simulink model "TST_RngMod_TrqFrcCalc"  (R2016b)
settings: Solver=FixedStepDiscrete  StartTime=0.0  StopTime=simTime  FixedStep=sampleTime  RelTol=1e-3
values from neighbouring files (symbols this model uses):
  testCase = 1    [initTST_RngMod_TrqFrcCalc_001.m]    (also in initTST_RngMod_TrqFrcCalc_002.m = 2; initTST_RngMod_TrqFrcCalc_003.m = 3)
libraries: simulink x4
settings Model: Creator=guofang02  LastModifiedBy=guofang02
settings ConfigComp: CovHTMLOptions=-sRT=0  CovHtmlReporting=on  CovSaveCumulativeToWorkspaceVar=on  CovCumulativeVarName=RngMod_TrqFrcCalc_covCumulativeData  CovCumulativeReport=on  CovShowResultsExplorer=off

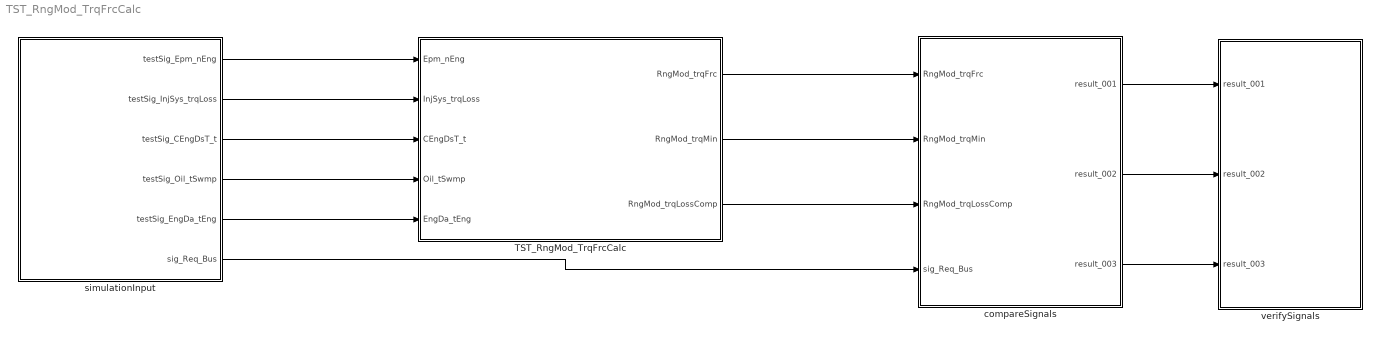
== system TST_RngMod_TrqFrcCalc ==
  TST_RngMod_TrqFrcCalc : Subsystem
  compareSignals : Subsystem
  simulationInput : Subsystem
  verifySignals : Subsystem
  wires:
  simulationInput/1(testSig_Epm_nEng) -> TST_RngMod_TrqFrcCalc/1(Epm_nEng)
  simulationInput/2(testSig_InjSys_trqLoss) -> TST_RngMod_TrqFrcCalc/2(InjSys_trqLoss)
  simulationInput/3(testSig_CEngDsT_t) -> TST_RngMod_TrqFrcCalc/3(CEngDsT_t)
  simulationInput/4(testSig_Oil_tSwmp) -> TST_RngMod_TrqFrcCalc/4(Oil_tSwmp)
  simulationInput/5(testSig_EngDa_tEng) -> TST_RngMod_TrqFrcCalc/5(EngDa_tEng)
  TST_RngMod_TrqFrcCalc/1(RngMod_trqFrc) -> compareSignals/1(RngMod_trqFrc)
  TST_RngMod_TrqFrcCalc/2(RngMod_trqMin) -> compareSignals/2(RngMod_trqMin)
  TST_RngMod_TrqFrcCalc/3(RngMod_trqLossComp) -> compareSignals/3(RngMod_trqLossComp)
  simulationInput/6(sig_Req_Bus) -> compareSignals/4(sig_Req_Bus)
  compareSignals/1(result_001) -> verifySignals/1(result_001)
  compareSignals/2(result_002) -> verifySignals/2(result_002)
  compareSignals/3(result_003) -> verifySignals/3(result_003)

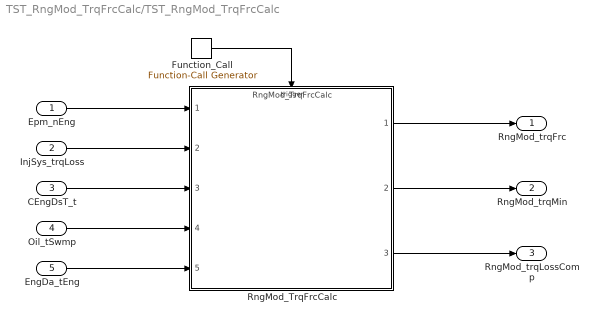
== system TST_RngMod_TrqFrcCalc/TST_RngMod_TrqFrcCalc ==
  Epm_nEng : Inport
  InjSys_trqLoss : Inport  Port=2
  CEngDsT_t : Inport  Port=3
  Oil_tSwmp : Inport  Port=4
  EngDa_tEng : Inport  Port=5
  Function_Call : simulink/Ports & Subsystems/Function-Call Generator  sample_time=sampleTime  numberOfIterations=1
  RngMod_TrqFrcCalc : ModelReference  ModelNameDialog=RngMod_TrqFrcCalc  SimulationMode=Normal  ModelReferenceVersion=1.4  TriggerPortName=function  TriggerPortTriggerType=function-call  TriggerPortStatesWhenEnabling=held
  RngMod_trqFrc : Outport
  RngMod_trqMin : Outport  Port=2
  RngMod_trqLossComp : Outport  Port=3
  wires:
  Function_Call/1 -> RngMod_TrqFrcCalc/Trigger
  Epm_nEng/1 -> RngMod_TrqFrcCalc/1
  InjSys_trqLoss/1 -> RngMod_TrqFrcCalc/2
  CEngDsT_t/1 -> RngMod_TrqFrcCalc/3
  Oil_tSwmp/1 -> RngMod_TrqFrcCalc/4
  EngDa_tEng/1 -> RngMod_TrqFrcCalc/5
  RngMod_TrqFrcCalc/1 -> RngMod_trqFrc/1
  RngMod_TrqFrcCalc/2 -> RngMod_trqMin/1
  RngMod_TrqFrcCalc/3 -> RngMod_trqLossComp/1

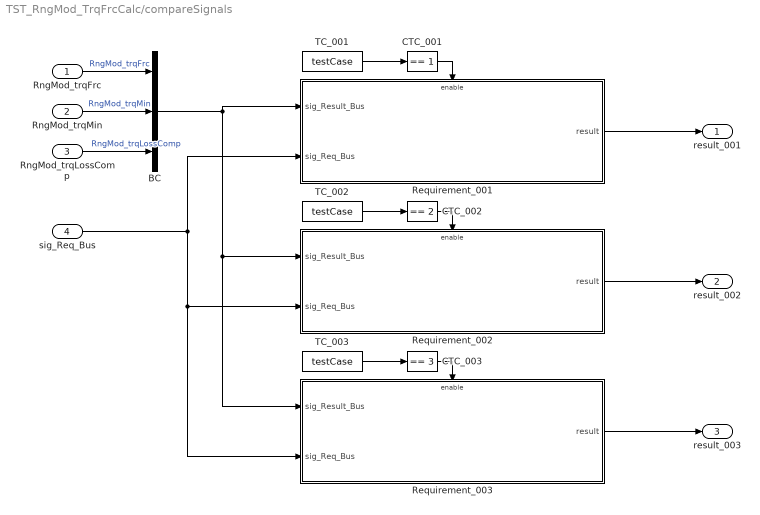
== system TST_RngMod_TrqFrcCalc/compareSignals ==
  RngMod_trqFrc : Inport
  RngMod_trqMin : Inport  Port=2
  RngMod_trqLossComp : Inport  Port=3
  sig_Req_Bus : Inport  Port=4
  BC : BusCreator  Inputs=3
  CTC_001 : simulink/Logic and Bit Operations/Compare To Constant  relop===  const=1  OutDataTypeStr=boolean
  CTC_002 : simulink/Logic and Bit Operations/Compare To Constant  relop===  const=2  OutDataTypeStr=boolean
  CTC_003 : simulink/Logic and Bit Operations/Compare To Constant  relop===  const=3  OutDataTypeStr=boolean
  Requirement_001 : Subsystem
  Requirement_002 : Subsystem
  Requirement_003 : Subsystem
  TC_001 : Constant  Value=testCase
  TC_002 : Constant  Value=testCase
  TC_003 : Constant  Value=testCase
  result_001 : Outport
  result_002 : Outport  Port=2
  result_003 : Outport  Port=3
  wires:
  RngMod_trqFrc/1 -> BC/1  "RngMod_trqFrc"
  RngMod_trqMin/1 -> BC/2  "RngMod_trqMin"
  RngMod_trqLossComp/1 -> BC/3  "RngMod_trqLossComp"
  TC_001/1 -> CTC_001/1
  CTC_001/1 -> Requirement_001/Enable
  sig_Req_Bus/1 -> Requirement_002/2(sig_Req_Bus), Requirement_003/2(sig_Req_Bus), Requirement_001/2(sig_Req_Bus)
  BC/1 -> Requirement_002/1(sig_Result_Bus), Requirement_003/1(sig_Result_Bus), Requirement_001/1(sig_Result_Bus)
  Requirement_001/1(result) -> result_001/1
  TC_002/1 -> CTC_002/1
  CTC_002/1 -> Requirement_002/Enable
  Requirement_002/1(result) -> result_002/1
  TC_003/1 -> CTC_003/1
  CTC_003/1 -> Requirement_003/Enable
  Requirement_003/1(result) -> result_003/1

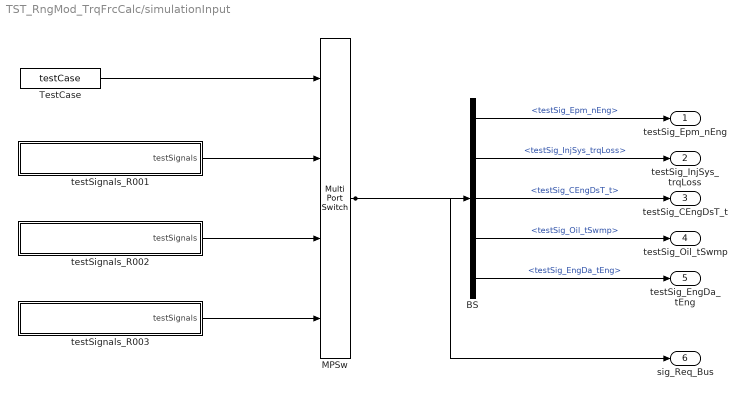
== system TST_RngMod_TrqFrcCalc/simulationInput ==
  BS : BusSelector  OutputSignals=testSig_Epm_nEng,testSig_InjSys_trqLoss,testSig_CEngDsT_t,testSig_Oil_tSwmp,testSig_EngDa_tEng
  MPSw : MultiPortSwitch  SaturateOnIntegerOverflow=on  InputSameDT=on
  TestCase : Constant  Value=testCase
  testSignals_R001 : Subsystem
  testSignals_R002 : Subsystem
  testSignals_R003 : Subsystem
  testSig_Epm_nEng : Outport
  testSig_InjSys_trqLoss : Outport  Port=2
  testSig_CEngDsT_t : Outport  Port=3
  testSig_Oil_tSwmp : Outport  Port=4
  testSig_EngDa_tEng : Outport  Port=5
  sig_Req_Bus : Outport  Port=6
  wires:
  BS/1 -> testSig_Epm_nEng/1  "<testSig_Epm_nEng>"
  BS/2 -> testSig_InjSys_trqLoss/1  "<testSig_InjSys_trqLoss>"
  BS/3 -> testSig_CEngDsT_t/1  "<testSig_CEngDsT_t>"
  BS/4 -> testSig_Oil_tSwmp/1  "<testSig_Oil_tSwmp>"
  BS/5 -> testSig_EngDa_tEng/1  "<testSig_EngDa_tEng>"
  MPSw/1 -> BS/1, sig_Req_Bus/1
  TestCase/1 -> MPSw/1
  testSignals_R001/1(testSignals) -> MPSw/2
  testSignals_R002/1(testSignals) -> MPSw/3
  testSignals_R003/1(testSignals) -> MPSw/4

== system TST_RngMod_TrqFrcCalc/verifySignals ==
  result_001 : Inport
  result_002 : Inport  Port=2
  result_003 : Inport  Port=3
  Assertion_001 : Assertion  Enabled=off
  Assertion_002 : Assertion  Enabled=off
  Assertion_003 : Assertion
  wires:
  result_001/1 -> Assertion_001/1
  result_002/1 -> Assertion_002/1
  result_003/1 -> Assertion_003/1

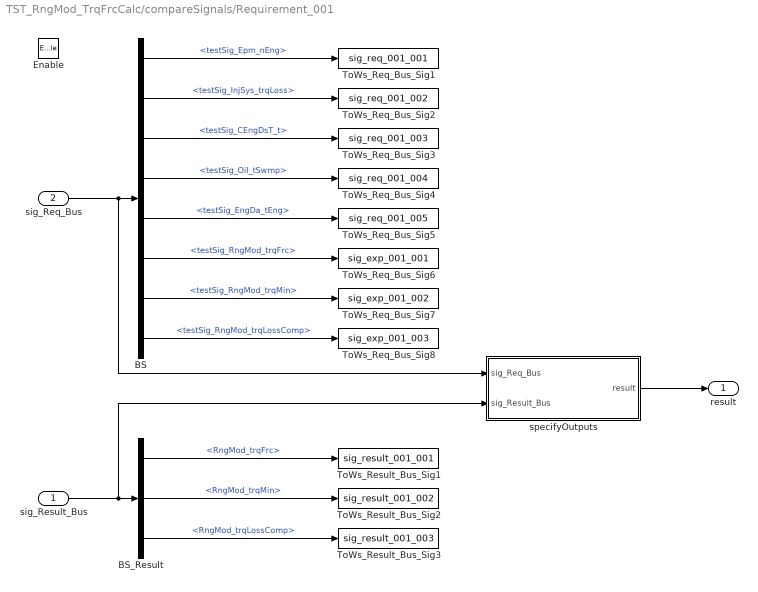
== system TST_RngMod_TrqFrcCalc/compareSignals/Requirement_001 ==
  sig_Result_Bus : Inport
  sig_Req_Bus : Inport  Port=2
  Enable : EnablePort
  BS : BusSelector  OutputSignals=testSig_Epm_nEng,testSig_InjSys_trqLoss,testSig_CEngDsT_t,testSig_Oil_tSwmp,testSig_EngDa_tEng,testSig_RngMod_trqFrc,testSig_RngMod_trqMin,testSig_RngMod_trqLossComp
  BS_Result : BusSelector  OutputSignals=RngMod_trqFrc,RngMod_trqMin,RngMod_trqLossComp
  ToWs_Req_Bus_Sig1 : ToWorkspace  VariableName=sig_req_001_001  SaveFormat=Structure With Time
  ToWs_Req_Bus_Sig2 : ToWorkspace  VariableName=sig_req_001_002  SaveFormat=Structure With Time
  ToWs_Req_Bus_Sig3 : ToWorkspace  VariableName=sig_req_001_003  SaveFormat=Structure With Time
  ToWs_Req_Bus_Sig4 : ToWorkspace  VariableName=sig_req_001_004  SaveFormat=Structure With Time
  ToWs_Req_Bus_Sig5 : ToWorkspace  VariableName=sig_req_001_005  SaveFormat=Structure With Time
  ToWs_Req_Bus_Sig6 : ToWorkspace  VariableName=sig_exp_001_001  SaveFormat=Structure With Time
  ToWs_Req_Bus_Sig7 : ToWorkspace  VariableName=sig_exp_001_002  SaveFormat=Structure With Time
  ToWs_Req_Bus_Sig8 : ToWorkspace  VariableName=sig_exp_001_003  SaveFormat=Structure With Time
  ToWs_Result_Bus_Sig1 : ToWorkspace  VariableName=sig_result_001_001  SaveFormat=Structure With Time
  ToWs_Result_Bus_Sig2 : ToWorkspace  VariableName=sig_result_001_002  SaveFormat=Structure With Time
  ToWs_Result_Bus_Sig3 : ToWorkspace  VariableName=sig_result_001_003  SaveFormat=Structure With Time
  specifyOutputs : Subsystem
  result : Outport
  wires:
  sig_Req_Bus/1 -> BS/1, specifyOutputs/1(sig_Req_Bus)
  BS/1 -> ToWs_Req_Bus_Sig1/1  "<testSig_Epm_nEng>"
  BS/2 -> ToWs_Req_Bus_Sig2/1  "<testSig_InjSys_trqLoss>"
  BS/3 -> ToWs_Req_Bus_Sig3/1  "<testSig_CEngDsT_t>"
  BS/4 -> ToWs_Req_Bus_Sig4/1  "<testSig_Oil_tSwmp>"
  BS/5 -> ToWs_Req_Bus_Sig5/1  "<testSig_EngDa_tEng>"
  BS/6 -> ToWs_Req_Bus_Sig6/1  "<testSig_RngMod_trqFrc>"
  BS/7 -> ToWs_Req_Bus_Sig7/1  "<testSig_RngMod_trqMin>"
  BS/8 -> ToWs_Req_Bus_Sig8/1  "<testSig_RngMod_trqLossComp>"
  sig_Result_Bus/1 -> BS_Result/1, specifyOutputs/2(sig_Result_Bus)
  BS_Result/1 -> ToWs_Result_Bus_Sig1/1  "<RngMod_trqFrc>"
  BS_Result/2 -> ToWs_Result_Bus_Sig2/1  "<RngMod_trqMin>"
  BS_Result/3 -> ToWs_Result_Bus_Sig3/1  "<RngMod_trqLossComp>"
  specifyOutputs/1(result) -> result/1

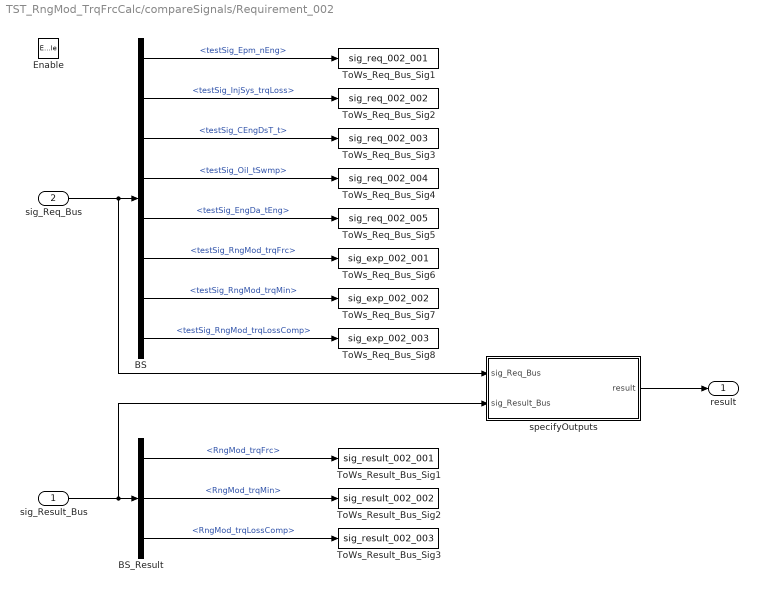
== system TST_RngMod_TrqFrcCalc/compareSignals/Requirement_002 ==
  sig_Result_Bus : Inport
  sig_Req_Bus : Inport  Port=2
  Enable : EnablePort
  BS : BusSelector  OutputSignals=testSig_Epm_nEng,testSig_InjSys_trqLoss,testSig_CEngDsT_t,testSig_Oil_tSwmp,testSig_EngDa_tEng,testSig_RngMod_trqFrc,testSig_RngMod_trqMin,testSig_RngMod_trqLossComp
  BS_Result : BusSelector  OutputSignals=RngMod_trqFrc,RngMod_trqMin,RngMod_trqLossComp
  ToWs_Req_Bus_Sig1 : ToWorkspace  VariableName=sig_req_002_001  SaveFormat=Structure With Time
  ToWs_Req_Bus_Sig2 : ToWorkspace  VariableName=sig_req_002_002  SaveFormat=Structure With Time
  ToWs_Req_Bus_Sig3 : ToWorkspace  VariableName=sig_req_002_003  SaveFormat=Structure With Time
  ToWs_Req_Bus_Sig4 : ToWorkspace  VariableName=sig_req_002_004  SaveFormat=Structure With Time
  ToWs_Req_Bus_Sig5 : ToWorkspace  VariableName=sig_req_002_005  SaveFormat=Structure With Time
  ToWs_Req_Bus_Sig6 : ToWorkspace  VariableName=sig_exp_002_001  SaveFormat=Structure With Time
  ToWs_Req_Bus_Sig7 : ToWorkspace  VariableName=sig_exp_002_002  SaveFormat=Structure With Time
  ToWs_Req_Bus_Sig8 : ToWorkspace  VariableName=sig_exp_002_003  SaveFormat=Structure With Time
  ToWs_Result_Bus_Sig1 : ToWorkspace  VariableName=sig_result_002_001  SaveFormat=Structure With Time
  ToWs_Result_Bus_Sig2 : ToWorkspace  VariableName=sig_result_002_002  SaveFormat=Structure With Time
  ToWs_Result_Bus_Sig3 : ToWorkspace  VariableName=sig_result_002_003  SaveFormat=Structure With Time
  specifyOutputs : Subsystem
  result : Outport
  wires:
  sig_Req_Bus/1 -> BS/1, specifyOutputs/1(sig_Req_Bus)
  BS/1 -> ToWs_Req_Bus_Sig1/1  "<testSig_Epm_nEng>"
  BS/2 -> ToWs_Req_Bus_Sig2/1  "<testSig_InjSys_trqLoss>"
  BS/3 -> ToWs_Req_Bus_Sig3/1  "<testSig_CEngDsT_t>"
  BS/4 -> ToWs_Req_Bus_Sig4/1  "<testSig_Oil_tSwmp>"
  BS/5 -> ToWs_Req_Bus_Sig5/1  "<testSig_EngDa_tEng>"
  BS/6 -> ToWs_Req_Bus_Sig6/1  "<testSig_RngMod_trqFrc>"
  BS/7 -> ToWs_Req_Bus_Sig7/1  "<testSig_RngMod_trqMin>"
  BS/8 -> ToWs_Req_Bus_Sig8/1  "<testSig_RngMod_trqLossComp>"
  sig_Result_Bus/1 -> BS_Result/1, specifyOutputs/2(sig_Result_Bus)
  BS_Result/1 -> ToWs_Result_Bus_Sig1/1  "<RngMod_trqFrc>"
  BS_Result/2 -> ToWs_Result_Bus_Sig2/1  "<RngMod_trqMin>"
  BS_Result/3 -> ToWs_Result_Bus_Sig3/1  "<RngMod_trqLossComp>"
  specifyOutputs/1(result) -> result/1

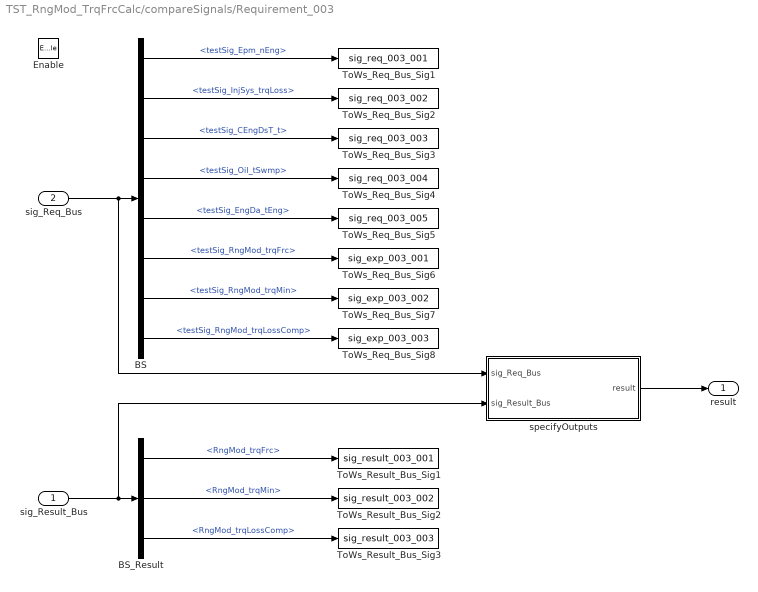
== system TST_RngMod_TrqFrcCalc/compareSignals/Requirement_003 ==
  sig_Result_Bus : Inport
  sig_Req_Bus : Inport  Port=2
  Enable : EnablePort
  BS : BusSelector  OutputSignals=testSig_Epm_nEng,testSig_InjSys_trqLoss,testSig_CEngDsT_t,testSig_Oil_tSwmp,testSig_EngDa_tEng,testSig_RngMod_trqFrc,testSig_RngMod_trqMin,testSig_RngMod_trqLossComp
  BS_Result : BusSelector  OutputSignals=RngMod_trqFrc,RngMod_trqMin,RngMod_trqLossComp
  ToWs_Req_Bus_Sig1 : ToWorkspace  VariableName=sig_req_003_001  SaveFormat=Structure With Time
  ToWs_Req_Bus_Sig2 : ToWorkspace  VariableName=sig_req_003_002  SaveFormat=Structure With Time
  ToWs_Req_Bus_Sig3 : ToWorkspace  VariableName=sig_req_003_003  SaveFormat=Structure With Time
  ToWs_Req_Bus_Sig4 : ToWorkspace  VariableName=sig_req_003_004  SaveFormat=Structure With Time
  ToWs_Req_Bus_Sig5 : ToWorkspace  VariableName=sig_req_003_005  SaveFormat=Structure With Time
  ToWs_Req_Bus_Sig6 : ToWorkspace  VariableName=sig_exp_003_001  SaveFormat=Structure With Time
  ToWs_Req_Bus_Sig7 : ToWorkspace  VariableName=sig_exp_003_002  SaveFormat=Structure With Time
  ToWs_Req_Bus_Sig8 : ToWorkspace  VariableName=sig_exp_003_003  SaveFormat=Structure With Time
  ToWs_Result_Bus_Sig1 : ToWorkspace  VariableName=sig_result_003_001  SaveFormat=Structure With Time
  ToWs_Result_Bus_Sig2 : ToWorkspace  VariableName=sig_result_003_002  SaveFormat=Structure With Time
  ToWs_Result_Bus_Sig3 : ToWorkspace  VariableName=sig_result_003_003  SaveFormat=Structure With Time
  specifyOutputs : Subsystem
  result : Outport
  wires:
  sig_Req_Bus/1 -> BS/1, specifyOutputs/1(sig_Req_Bus)
  BS/1 -> ToWs_Req_Bus_Sig1/1  "<testSig_Epm_nEng>"
  BS/2 -> ToWs_Req_Bus_Sig2/1  "<testSig_InjSys_trqLoss>"
  BS/3 -> ToWs_Req_Bus_Sig3/1  "<testSig_CEngDsT_t>"
  BS/4 -> ToWs_Req_Bus_Sig4/1  "<testSig_Oil_tSwmp>"
  BS/5 -> ToWs_Req_Bus_Sig5/1  "<testSig_EngDa_tEng>"
  BS/6 -> ToWs_Req_Bus_Sig6/1  "<testSig_RngMod_trqFrc>"
  BS/7 -> ToWs_Req_Bus_Sig7/1  "<testSig_RngMod_trqMin>"
  BS/8 -> ToWs_Req_Bus_Sig8/1  "<testSig_RngMod_trqLossComp>"
  sig_Result_Bus/1 -> BS_Result/1, specifyOutputs/2(sig_Result_Bus)
  BS_Result/1 -> ToWs_Result_Bus_Sig1/1  "<RngMod_trqFrc>"
  BS_Result/2 -> ToWs_Result_Bus_Sig2/1  "<RngMod_trqMin>"
  BS_Result/3 -> ToWs_Result_Bus_Sig3/1  "<RngMod_trqLossComp>"
  specifyOutputs/1(result) -> result/1

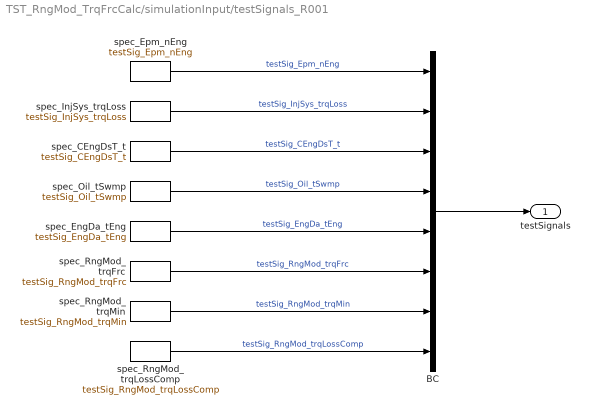
== system TST_RngMod_TrqFrcCalc/simulationInput/testSignals_R001 ==
  BC : BusCreator  Inputs=8
  spec_CEngDsT_t : FromWorkspace  VariableName=testSig_CEngDsT_t  Interpolate=off  OutputAfterFinalValue=Holding final value
  spec_EngDa_tEng : FromWorkspace  VariableName=testSig_EngDa_tEng  Interpolate=off  OutputAfterFinalValue=Holding final value
  spec_Epm_nEng : FromWorkspace  VariableName=testSig_Epm_nEng  Interpolate=off  OutputAfterFinalValue=Holding final value
  spec_InjSys_trqLoss : FromWorkspace  VariableName=testSig_InjSys_trqLoss  Interpolate=off  OutputAfterFinalValue=Holding final value
  spec_Oil_tSwmp : FromWorkspace  VariableName=testSig_Oil_tSwmp  Interpolate=off  OutputAfterFinalValue=Holding final value
  spec_RngMod_trqFrc : FromWorkspace  VariableName=testSig_RngMod_trqFrc  Interpolate=off  OutputAfterFinalValue=Holding final value
  spec_RngMod_trqLossComp : FromWorkspace  VariableName=testSig_RngMod_trqLossComp  Interpolate=off  OutputAfterFinalValue=Holding final value
  spec_RngMod_trqMin : FromWorkspace  VariableName=testSig_RngMod_trqMin  Interpolate=off  OutputAfterFinalValue=Holding final value
  testSignals : Outport
  wires:
  BC/1 -> testSignals/1
  spec_Epm_nEng/1 -> BC/1  "testSig_Epm_nEng"
  spec_InjSys_trqLoss/1 -> BC/2  "testSig_InjSys_trqLoss"
  spec_CEngDsT_t/1 -> BC/3  "testSig_CEngDsT_t"
  spec_Oil_tSwmp/1 -> BC/4  "testSig_Oil_tSwmp"
  spec_EngDa_tEng/1 -> BC/5  "testSig_EngDa_tEng"
  spec_RngMod_trqFrc/1 -> BC/6  "testSig_RngMod_trqFrc"
  spec_RngMod_trqMin/1 -> BC/7  "testSig_RngMod_trqMin"
  spec_RngMod_trqLossComp/1 -> BC/8  "testSig_RngMod_trqLossComp"

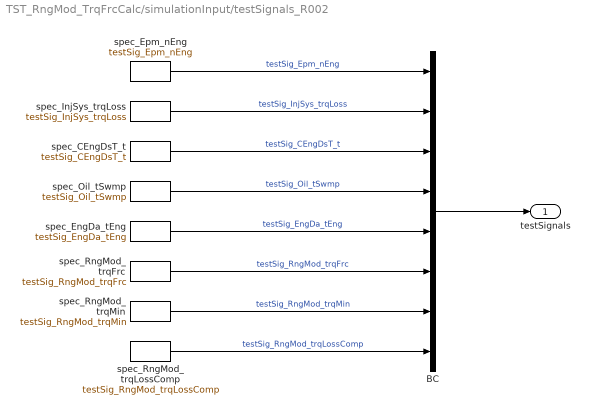
== system TST_RngMod_TrqFrcCalc/simulationInput/testSignals_R002 ==
  BC : BusCreator  Inputs=8
  spec_CEngDsT_t : FromWorkspace  VariableName=testSig_CEngDsT_t  Interpolate=off  OutputAfterFinalValue=Holding final value
  spec_EngDa_tEng : FromWorkspace  VariableName=testSig_EngDa_tEng  Interpolate=off  OutputAfterFinalValue=Holding final value
  spec_Epm_nEng : FromWorkspace  VariableName=testSig_Epm_nEng  Interpolate=off  OutputAfterFinalValue=Holding final value
  spec_InjSys_trqLoss : FromWorkspace  VariableName=testSig_InjSys_trqLoss  Interpolate=off  OutputAfterFinalValue=Holding final value
  spec_Oil_tSwmp : FromWorkspace  VariableName=testSig_Oil_tSwmp  Interpolate=off  OutputAfterFinalValue=Holding final value
  spec_RngMod_trqFrc : FromWorkspace  VariableName=testSig_RngMod_trqFrc  Interpolate=off  OutputAfterFinalValue=Holding final value
  spec_RngMod_trqLossComp : FromWorkspace  VariableName=testSig_RngMod_trqLossComp  Interpolate=off  OutputAfterFinalValue=Holding final value
  spec_RngMod_trqMin : FromWorkspace  VariableName=testSig_RngMod_trqMin  Interpolate=off  OutputAfterFinalValue=Holding final value
  testSignals : Outport
  wires:
  BC/1 -> testSignals/1
  spec_Epm_nEng/1 -> BC/1  "testSig_Epm_nEng"
  spec_InjSys_trqLoss/1 -> BC/2  "testSig_InjSys_trqLoss"
  spec_CEngDsT_t/1 -> BC/3  "testSig_CEngDsT_t"
  spec_Oil_tSwmp/1 -> BC/4  "testSig_Oil_tSwmp"
  spec_EngDa_tEng/1 -> BC/5  "testSig_EngDa_tEng"
  spec_RngMod_trqFrc/1 -> BC/6  "testSig_RngMod_trqFrc"
  spec_RngMod_trqMin/1 -> BC/7  "testSig_RngMod_trqMin"
  spec_RngMod_trqLossComp/1 -> BC/8  "testSig_RngMod_trqLossComp"

== system TST_RngMod_TrqFrcCalc/simulationInput/testSignals_R003 ==
  BC : BusCreator  Inputs=8
  spec_CEngDsT_t : FromWorkspace  VariableName=testSig_CEngDsT_t  Interpolate=off  OutputAfterFinalValue=Holding final value
  spec_EngDa_tEng : FromWorkspace  VariableName=testSig_EngDa_tEng  Interpolate=off  OutputAfterFinalValue=Holding final value
  spec_Epm_nEng : FromWorkspace  VariableName=testSig_Epm_nEng  Interpolate=off  OutputAfterFinalValue=Holding final value
  spec_InjSys_trqLoss : FromWorkspace  VariableName=testSig_InjSys_trqLoss  Interpolate=off  OutputAfterFinalValue=Holding final value
  spec_Oil_tSwmp : FromWorkspace  VariableName=testSig_Oil_tSwmp  Interpolate=off  OutputAfterFinalValue=Holding final value
  spec_RngMod_trqFrc : FromWorkspace  VariableName=testSig_RngMod_trqFrc  Interpolate=off  OutputAfterFinalValue=Holding final value
  spec_RngMod_trqLossComp : FromWorkspace  VariableName=testSig_RngMod_trqLossComp  Interpolate=off  OutputAfterFinalValue=Holding final value
  spec_RngMod_trqMin : FromWorkspace  VariableName=testSig_RngMod_trqMin  Interpolate=off  OutputAfterFinalValue=Holding final value
  testSignals : Outport
  wires:
  BC/1 -> testSignals/1
  spec_Epm_nEng/1 -> BC/1  "testSig_Epm_nEng"
  spec_InjSys_trqLoss/1 -> BC/2  "testSig_InjSys_trqLoss"
  spec_CEngDsT_t/1 -> BC/3  "testSig_CEngDsT_t"
  spec_Oil_tSwmp/1 -> BC/4  "testSig_Oil_tSwmp"
  spec_EngDa_tEng/1 -> BC/5  "testSig_EngDa_tEng"
  spec_RngMod_trqFrc/1 -> BC/6  "testSig_RngMod_trqFrc"
  spec_RngMod_trqMin/1 -> BC/7  "testSig_RngMod_trqMin"
  spec_RngMod_trqLossComp/1 -> BC/8  "testSig_RngMod_trqLossComp"

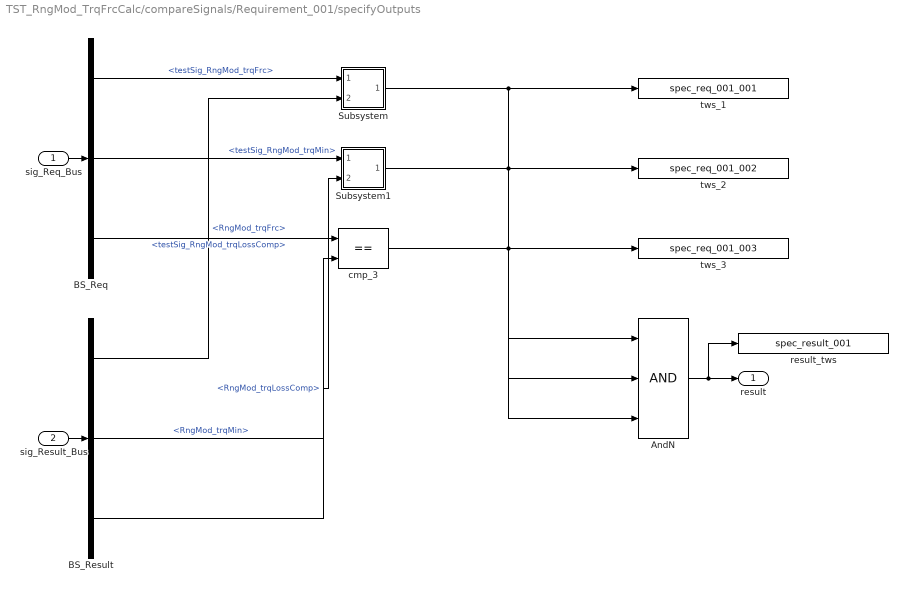
== system TST_RngMod_TrqFrcCalc/compareSignals/Requirement_001/specifyOutputs ==
  sig_Req_Bus : Inport
  sig_Result_Bus : Inport  Port=2
  AndN : Logic  Inputs=3
  BS_Req : BusSelector  OutputSignals=testSig_RngMod_trqFrc,testSig_RngMod_trqMin,testSig_RngMod_trqLossComp
  BS_Result : BusSelector  OutputSignals=RngMod_trqFrc,RngMod_trqMin,RngMod_trqLossComp
  Subsystem : Subsystem
  Subsystem1 : Subsystem
  cmp_3 : RelationalOperator  Operator===  RndMeth=Nearest  InputSameDT=on
  result_tws : ToWorkspace  VariableName=spec_result_001
  tws_1 : ToWorkspace  VariableName=spec_req_001_001
  tws_2 : ToWorkspace  VariableName=spec_req_001_002
  tws_3 : ToWorkspace  VariableName=spec_req_001_003
  result : Outport
  wires:
  sig_Req_Bus/1 -> BS_Req/1
  sig_Result_Bus/1 -> BS_Result/1
  AndN/1 -> result/1, result_tws/1
  BS_Req/1 -> Subsystem/1(In1)  "<testSig_RngMod_trqFrc>"
  BS_Result/1 -> Subsystem/2(In2)  "<RngMod_trqFrc>"
  Subsystem/1(Out1) -> tws_1/1, AndN/1
  BS_Req/2 -> Subsystem1/1(In1)  "<testSig_RngMod_trqMin>"
  BS_Result/2 -> Subsystem1/2(In2)  "<RngMod_trqMin>"
  Subsystem1/1(Out1) -> tws_2/1, AndN/2
  BS_Req/3 -> cmp_3/1  "<testSig_RngMod_trqLossComp>"
  BS_Result/3 -> cmp_3/2  "<RngMod_trqLossComp>"
  cmp_3/1 -> tws_3/1, AndN/3

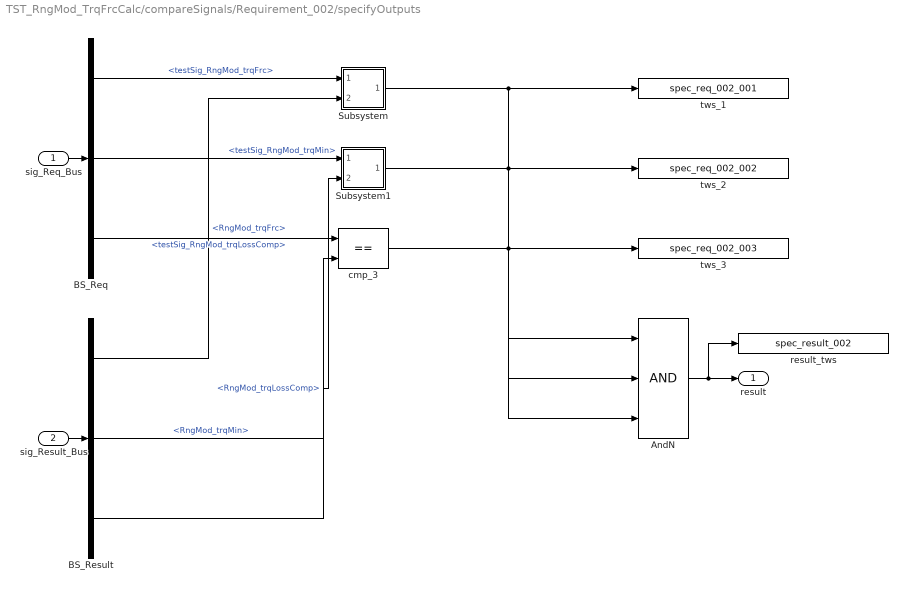
== system TST_RngMod_TrqFrcCalc/compareSignals/Requirement_002/specifyOutputs ==
  sig_Req_Bus : Inport
  sig_Result_Bus : Inport  Port=2
  AndN : Logic  Inputs=3
  BS_Req : BusSelector  OutputSignals=testSig_RngMod_trqFrc,testSig_RngMod_trqMin,testSig_RngMod_trqLossComp
  BS_Result : BusSelector  OutputSignals=RngMod_trqFrc,RngMod_trqMin,RngMod_trqLossComp
  Subsystem : Subsystem
  Subsystem1 : Subsystem
  cmp_3 : RelationalOperator  Operator===  RndMeth=Nearest  InputSameDT=on
  result_tws : ToWorkspace  VariableName=spec_result_002
  tws_1 : ToWorkspace  VariableName=spec_req_002_001
  tws_2 : ToWorkspace  VariableName=spec_req_002_002
  tws_3 : ToWorkspace  VariableName=spec_req_002_003
  result : Outport
  wires:
  sig_Req_Bus/1 -> BS_Req/1
  sig_Result_Bus/1 -> BS_Result/1
  AndN/1 -> result/1, result_tws/1
  BS_Req/1 -> Subsystem/1(In1)  "<testSig_RngMod_trqFrc>"
  BS_Result/1 -> Subsystem/2(In2)  "<RngMod_trqFrc>"
  Subsystem/1(Out1) -> tws_1/1, AndN/1
  BS_Req/2 -> Subsystem1/1(In1)  "<testSig_RngMod_trqMin>"
  BS_Result/2 -> Subsystem1/2(In2)  "<RngMod_trqMin>"
  Subsystem1/1(Out1) -> tws_2/1, AndN/2
  BS_Req/3 -> cmp_3/1  "<testSig_RngMod_trqLossComp>"
  BS_Result/3 -> cmp_3/2  "<RngMod_trqLossComp>"
  cmp_3/1 -> tws_3/1, AndN/3

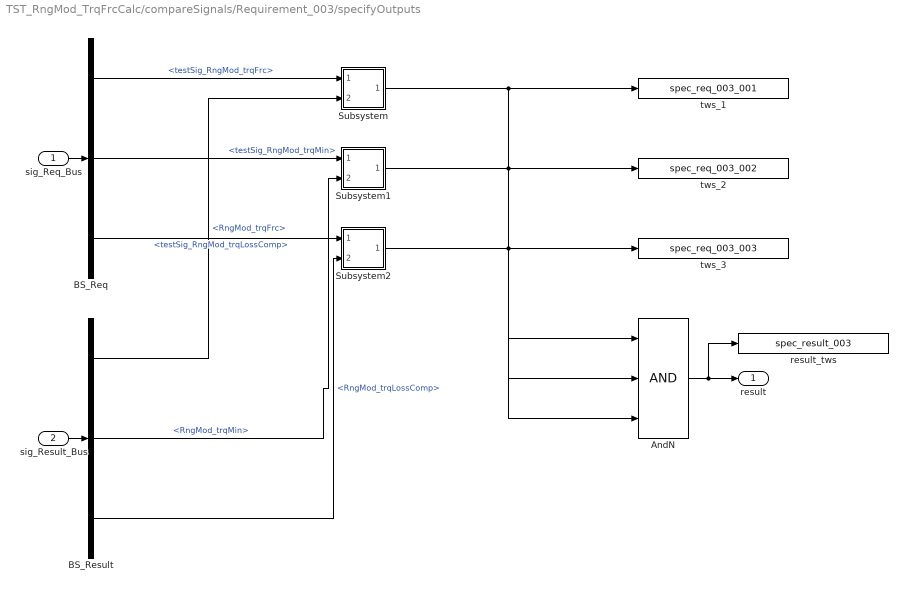
== system TST_RngMod_TrqFrcCalc/compareSignals/Requirement_003/specifyOutputs ==
  sig_Req_Bus : Inport
  sig_Result_Bus : Inport  Port=2
  AndN : Logic  Inputs=3
  BS_Req : BusSelector  OutputSignals=testSig_RngMod_trqFrc,testSig_RngMod_trqMin,testSig_RngMod_trqLossComp
  BS_Result : BusSelector  OutputSignals=RngMod_trqFrc,RngMod_trqMin,RngMod_trqLossComp
  Subsystem : Subsystem
  Subsystem1 : Subsystem
  Subsystem2 : Subsystem
  result_tws : ToWorkspace  VariableName=spec_result_003
  tws_1 : ToWorkspace  VariableName=spec_req_003_001
  tws_2 : ToWorkspace  VariableName=spec_req_003_002
  tws_3 : ToWorkspace  VariableName=spec_req_003_003
  result : Outport
  wires:
  sig_Req_Bus/1 -> BS_Req/1
  sig_Result_Bus/1 -> BS_Result/1
  AndN/1 -> result/1, result_tws/1
  BS_Req/1 -> Subsystem/1(In1)  "<testSig_RngMod_trqFrc>"
  BS_Result/1 -> Subsystem/2(In2)  "<RngMod_trqFrc>"
  Subsystem/1(Out1) -> tws_1/1, AndN/1
  BS_Req/2 -> Subsystem1/1(In1)  "<testSig_RngMod_trqMin>"
  BS_Result/2 -> Subsystem1/2(In2)  "<RngMod_trqMin>"
  Subsystem1/1(Out1) -> tws_2/1, AndN/2
  BS_Req/3 -> Subsystem2/1(In1)  "<testSig_RngMod_trqLossComp>"
  BS_Result/3 -> Subsystem2/2(In2)  "<RngMod_trqLossComp>"
  Subsystem2/1(Out1) -> tws_3/1, AndN/3

== system TST_RngMod_TrqFrcCalc/compareSignals/Requirement_001/specifyOutputs/Subsystem ==
  In1 : Inport
  In2 : Inport  Port=2
  Abs : Abs
  Add : Sum  Inputs=+-
  Constant : Constant  Value=0.1
  Data Type Conversion : DataTypeConversion
  Relational Operator : RelationalOperator  Operator=<=  OutDataTypeStr=boolean  RndMeth=Simplest
  Out1 : Outport
  wires:
  In1/1 -> Add/1
  In2/1 -> Add/2
  Constant/1 -> Data Type Conversion/1
  Add/1 -> Abs/1
  Data Type Conversion/1 -> Relational Operator/2
  Relational Operator/1 -> Out1/1
  Abs/1 -> Relational Operator/1

== system TST_RngMod_TrqFrcCalc/compareSignals/Requirement_001/specifyOutputs/Subsystem1 ==
  In1 : Inport
  In2 : Inport  Port=2
  Abs : Abs
  Add : Sum  Inputs=+-
  Constant : Constant  Value=0.1
  Data Type Conversion : DataTypeConversion
  Relational Operator : RelationalOperator  Operator=<=  OutDataTypeStr=boolean  RndMeth=Simplest
  Out1 : Outport
  wires:
  In1/1 -> Add/1
  In2/1 -> Add/2
  Constant/1 -> Data Type Conversion/1
  Add/1 -> Abs/1
  Data Type Conversion/1 -> Relational Operator/2
  Relational Operator/1 -> Out1/1
  Abs/1 -> Relational Operator/1

== system TST_RngMod_TrqFrcCalc/compareSignals/Requirement_002/specifyOutputs/Subsystem ==
  In1 : Inport
  In2 : Inport  Port=2
  Abs : Abs
  Add : Sum  Inputs=+-
  Constant : Constant  Value=0.1
  Data Type Conversion : DataTypeConversion
  Relational Operator : RelationalOperator  Operator=<=  OutDataTypeStr=boolean  RndMeth=Simplest
  Out1 : Outport
  wires:
  In1/1 -> Add/1
  In2/1 -> Add/2
  Constant/1 -> Data Type Conversion/1
  Add/1 -> Abs/1
  Data Type Conversion/1 -> Relational Operator/2
  Relational Operator/1 -> Out1/1
  Abs/1 -> Relational Operator/1

== system TST_RngMod_TrqFrcCalc/compareSignals/Requirement_002/specifyOutputs/Subsystem1 ==
  In1 : Inport
  In2 : Inport  Port=2
  Abs : Abs
  Add : Sum  Inputs=+-
  Constant : Constant  Value=0.1
  Data Type Conversion : DataTypeConversion
  Relational Operator : RelationalOperator  Operator=<=  OutDataTypeStr=boolean  RndMeth=Simplest
  Out1 : Outport
  wires:
  In1/1 -> Add/1
  In2/1 -> Add/2
  Constant/1 -> Data Type Conversion/1
  Add/1 -> Abs/1
  Data Type Conversion/1 -> Relational Operator/2
  Relational Operator/1 -> Out1/1
  Abs/1 -> Relational Operator/1

== system TST_RngMod_TrqFrcCalc/compareSignals/Requirement_003/specifyOutputs/Subsystem ==
  In1 : Inport
  In2 : Inport  Port=2
  Abs : Abs
  Add : Sum  Inputs=+-
  Constant : Constant  Value=0.1
  Data Type Conversion : DataTypeConversion
  Relational Operator : RelationalOperator  Operator=<=  OutDataTypeStr=boolean  RndMeth=Simplest
  Out1 : Outport
  wires:
  In1/1 -> Add/1
  In2/1 -> Add/2
  Constant/1 -> Data Type Conversion/1
  Add/1 -> Abs/1
  Data Type Conversion/1 -> Relational Operator/2
  Relational Operator/1 -> Out1/1
  Abs/1 -> Relational Operator/1

== system TST_RngMod_TrqFrcCalc/compareSignals/Requirement_003/specifyOutputs/Subsystem1 ==
  In1 : Inport
  In2 : Inport  Port=2
  Abs : Abs
  Add : Sum  Inputs=+-
  Constant : Constant  Value=0.1
  Data Type Conversion : DataTypeConversion
  Relational Operator : RelationalOperator  Operator=<=  OutDataTypeStr=boolean  RndMeth=Simplest
  Out1 : Outport
  wires:
  In1/1 -> Add/1
  In2/1 -> Add/2
  Constant/1 -> Data Type Conversion/1
  Add/1 -> Abs/1
  Data Type Conversion/1 -> Relational Operator/2
  Relational Operator/1 -> Out1/1
  Abs/1 -> Relational Operator/1

== system TST_RngMod_TrqFrcCalc/compareSignals/Requirement_003/specifyOutputs/Subsystem2 ==
  In1 : Inport
  In2 : Inport  Port=2
  Abs : Abs
  Add : Sum  Inputs=+-
  Constant : Constant  Value=0.1
  Data Type Conversion : DataTypeConversion
  Relational Operator : RelationalOperator  Operator=<=  OutDataTypeStr=boolean  RndMeth=Simplest
  Out1 : Outport
  wires:
  In1/1 -> Add/1
  In2/1 -> Add/2
  Constant/1 -> Data Type Conversion/1
  Add/1 -> Abs/1
  Data Type Conversion/1 -> Relational Operator/2
  Relational Operator/1 -> Out1/1
  Abs/1 -> Relational Operator/1
